simulink model "conttrolled_full_wave_rectification"  (R2024b)
settings: Solver=VariableStepAuto  StartTime=0.0  StopTime=10.0  MaxStep=1e-4  RelTol=1e-3
undefined symbols (not defined in the file or in its folder): alpha
libraries: spsThyristorLib x8, spsVoltageMeasurementLib x3, spsACVoltageSourceLib x2, spsMeanLib x2, spsSeriesRLCBranchLib x2, sps_lib x1
settings Model: Creator=Admin  LastModifiedBy=pragy

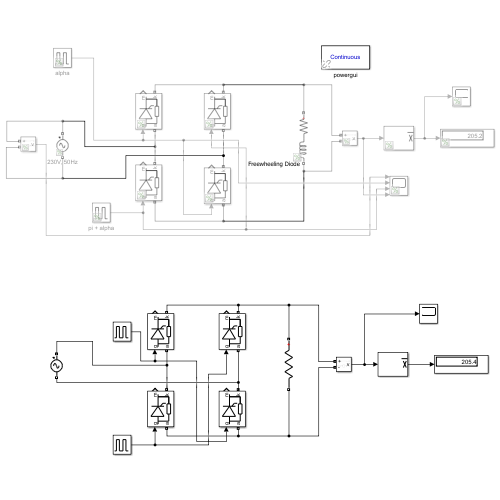
[thumbnail: Simulink's stored preview of the top-level diagram]
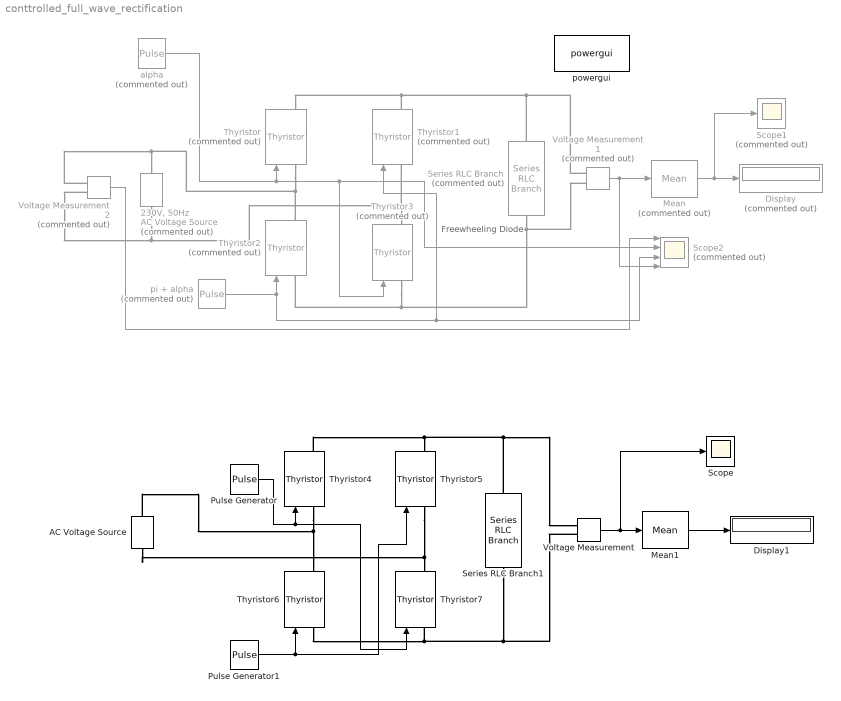
== system conttrolled_full_wave_rectification ==
  note: Freewheeling Diode
  "230V, 50Hz" : spsACVoltageSourceLib/AC Voltage Source  Commented=on  Amplitude=sqrt(2)*230  Phase=0  Frequency=50  SampleTime=0  Measurements=None  BusType=swing  Pref=10e3  Qref=0  Qmin=-inf  Qmax=+inf
  AC Voltage Source : spsACVoltageSourceLib/AC Voltage Source  Amplitude=230*sqrt(2)  Phase=0  Frequency=50  SampleTime=0  Measurements=None  BusType=swing  Pref=10e3  Qref=0  Qmin=-inf  Qmax=+inf
  Display : Display  Commented=on
  Display1 : Display
  Mean : spsMeanLib/Mean  Commented=on  Freq=50  Vinit=0  Ts=0
  Mean1 : spsMeanLib/Mean  Freq=50  Vinit=0  Ts=0
  Pulse Generator : DiscretePulseGenerator  PulseType=Time based  Period=1/50  PulseWidth=5  PhaseDelay=0*(0.02/360)
  Pulse Generator1 : DiscretePulseGenerator  PulseType=Time based  Period=1/50  PulseWidth=5  PhaseDelay=(0+180)*(0.02/360)
  Scope : Scope
  Scope1 : Scope  Commented=on
  Scope2 : Scope  Commented=on  NumInputPorts=4
  Series RLC Branch : spsSeriesRLCBranchLib/Series RLC Branch  Commented=on  LConnTagsString=__new0  RConnTagsString=__new0  BranchType=RL  Resistance=1.5  Inductance=1000e-3  SetiL0=off  InitialCurrent=0  Capacitance=1e-6  Setx0=off  InitialVoltage=0  Measurements=None
  Series RLC Branch1 : spsSeriesRLCBranchLib/Series RLC Branch  LConnTagsString=__new0  RConnTagsString=__new0  BranchType=R  Resistance=10  Inductance=1e-3  SetiL0=off  InitialCurrent=0  Capacitance=1e-6  Setx0=off  InitialVoltage=0  Measurements=None
  Thyristor{,1..3} (4 alike) : spsThyristorLib/Thyristor  Commented=on  Ron=0.001  Lon=0  Vf=0.8  IC=0  Rs=500  Cs=250e-9  Measurements=on
  Thyristor{4..7} (4 alike) : spsThyristorLib/Thyristor  Ron=0.001  Lon=0  Vf=0.8  IC=0  Rs=500  Cs=250e-9  Measurements=on
  Voltage Measurement : spsVoltageMeasurementLib/Voltage Measurement  PhasorSimulation=off  OutputType=Complex  PSBequivalent=0
  Voltage Measurement1 : spsVoltageMeasurementLib/Voltage Measurement  Commented=on  PhasorSimulation=off  OutputType=Complex  PSBequivalent=0
  Voltage Measurement2 : spsVoltageMeasurementLib/Voltage Measurement  Commented=on  PhasorSimulation=off  OutputType=Complex  PSBequivalent=0
  alpha : DiscretePulseGenerator  Commented=on  PulseType=Time based  Period=1/50  PulseWidth=5  PhaseDelay=(0.02/360)*alpha
  pi + alpha : DiscretePulseGenerator  Commented=on  PulseType=Time based  Period=1/50  PulseWidth=5  PhaseDelay=(0.02/360)*(180+alpha)
  powergui : sps_lib/powergui  Priority=1  SimulationMode=Continuous  SampleTime=50e-6  frequency=60  Iterations=50  frequencyindice=50  Pbase=100e6  ErrMax=1e-4  UnitsV=kV  UnitsW=MW  buscounter=0  FunctionMessages=off  echomessages=off  EnableUseOfTLC=off  CurrentSourceSwitches=off  DisableSnubberDevices=off  DisableRonSwitches=off  DisableVfSwitches=off  DisplayEquations=off  AutomaticDiscreteSolvers=off  SolverType=Tustin/Backward Euler (TBE)  Interpol=off  ExternalGateDelay=off  methode=off  Ts=100  x0status=zero  SPID=on  SwTol=0  HookPort=off  NonlinearTolerance=1e-4  nMaxIteration=100  ContinueOnMaxIteration=off  RestoreLinks=warning  ResistiveCurrentMeasurement=off  Frange=[0:2:500]  Ylog=off  Xlog=on  ShowGrid=off  save=off  variable=ZData  structure=0  ZoomFFT=off  StartTime=0.0  cycles=1  DisplayStyle=1  fundamental=60  FreqAxis=off  MaxFrequency=1000  frequencyindicesteady=1  RmsSteady=1  display=off
  wires:
  Voltage Measurement1/1 -> Scope2/4, Mean/1
  alpha/1 -> Thyristor3/1, Scope2/2, Thyristor/1
  pi + alpha/1 -> Thyristor1/1, Scope2/3, Thyristor2/1
  Mean/1 -> Display/1, Scope1/1
  Voltage Measurement2/1 -> Scope2/1
  Pulse Generator/1 -> Thyristor7/1, Thyristor4/1
  Pulse Generator1/1 -> Thyristor6/1, Thyristor5/1
  Voltage Measurement/1 -> Mean1/1, Scope/1
  Mean1/1 -> Display1/1
  connections:
  Voltage Measurement1/LConn2 -- Series RLC Branch/RConn1 -- Thyristor3/LConn1 -- Thyristor2/LConn1
  Voltage Measurement1/LConn1 -- Series RLC Branch/LConn1 -- Thyristor1/RConn1 -- Thyristor/RConn1
  Thyristor/LConn1 -- Thyristor2/RConn1 -- Voltage Measurement2/LConn1 -- "230V, 50Hz"/RConn1
  "230V, 50Hz"/LConn1 -- Voltage Measurement2/LConn2 -- Thyristor3/RConn1 -- Thyristor1/LConn1
  Thyristor4/LConn1 -- AC Voltage Source/RConn1 -- Thyristor6/RConn1
  Thyristor4/RConn1 -- Series RLC Branch1/LConn1 -- Voltage Measurement/LConn1 -- Thyristor5/RConn1
  Thyristor6/LConn1 -- Voltage Measurement/LConn2 -- Series RLC Branch1/RConn1 -- Thyristor7/LConn1
  Thyristor5/LConn1 -- AC Voltage Source/LConn1 -- Thyristor7/RConn1
